simulink model "Prac7_simu"  (R2025b)
settings: Solver=ode45  StartTime=0.0  StopTime=10.0  RelTol=1e-3
values from neighbouring files (symbols this model uses):
  b = 0.0012    [Prac7.m]
  J = 0.001    [Prac7.m]
  Ke = 0.01    [Prac7.m]
  Kt = Ke    (= 0.01)    [Prac7.m]
  La = 0.023    [Prac7.m]
  Ra = 2    [Prac7.m]
  T = 0    [Prac7.m]
settings Model: Creator=andre
settings RTWCC: GPUComputeCapability=3.5

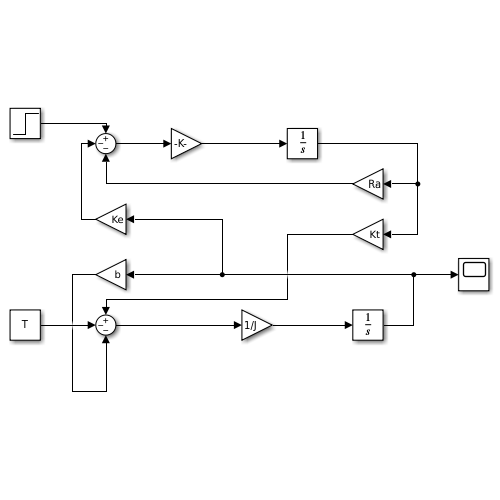
[thumbnail: Simulink's stored preview of the top-level diagram]
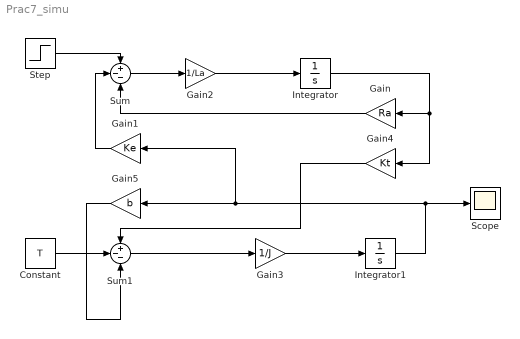
== system Prac7_simu ==
  Constant : Constant  Value=T
  Gain : Gain  Gain=Ra
  Gain1 : Gain  Gain=Ke
  Gain2 : Gain  Gain=1/La
  Gain3 : Gain  Gain=1/J
  Gain4 : Gain  Gain=Kt
  Gain5 : Gain  Gain=b
  Integrator : Integrator
  Integrator1 : Integrator
  Scope : Scope
      settings: ActiveDisplayYMinimum=-2.5000247365856434  ActiveDisplayYMaximum=22.500222629270795
  Step : Step  Time=0  After=5  SampleTime=0
  Sum : Sum  Inputs=+--
  Sum1 : Sum  Inputs=+--
  wires:
  Step/1 -> Sum/1
  Integrator/1 -> Gain4/1, Gain/1
  Gain/1 -> Sum/3
  Gain1/1 -> Sum/2
  Sum/1 -> Gain2/1
  Gain2/1 -> Integrator/1
  Gain3/1 -> Integrator1/1
  Sum1/1 -> Gain3/1
  Gain4/1 -> Sum1/1
  Constant/1 -> Sum1/2
  Gain5/1 -> Sum1/3
  Integrator1/1 -> Scope/1, Gain1/1, Gain5/1
